simulink model "hw9"  (R2020b)
settings: Solver=ode45  StartTime=0.0  StopTime=15  RelTol=1e-3
undefined symbols (not defined in the file or in its folder): controller, P, trajectory
settings Model: Creator=User  LastModifiedBy=User
settings DataIOCC: SaveFormat=Array  ReturnWorkspaceOutputs=off

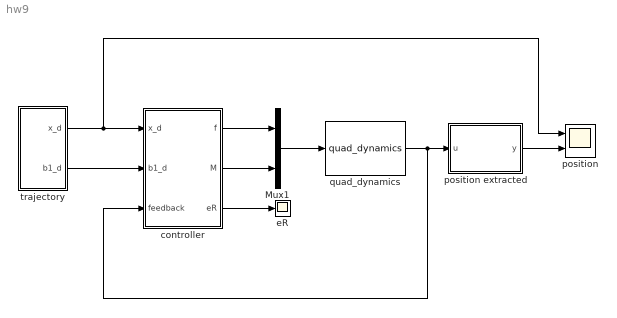
== system hw9 ==
  Mux1 : Mux  Inputs=2
  controller : Subsystem
  eR : Scope
  position : Scope  NumInputPorts=2
  position extracted : MATLAB Function  TreatAsAtomicUnit=on
  quad_dynamics : S-Function  FunctionName=quad_dynamics  Parameters=P  SFunctionDeploymentMode=off  EnableBusSupport=off
  trajectory : Subsystem
  wires:
  Mux1/1 -> quad_dynamics/1
  quad_dynamics/1 -> position extracted/1(u), controller/3(feedback)
  controller/1(f) -> Mux1/1
  controller/2(M) -> Mux1/2
  controller/3(eR) -> eR/1
  trajectory/1(x_d) -> controller/1(x_d), position/1
  trajectory/2(b1_d) -> controller/2(b1_d)
  position extracted/1(y) -> position/2

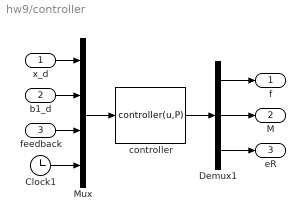
== system hw9/controller ==
  x_d : Inport
  b1_d : Inport  Port=2
  feedback : Inport  Port=3
  Clock1 : Clock
  Demux1 : Demux  Outputs=3
  Mux : Mux
  controller : MATLABFcn  MATLABFcn=controller(u,P)  OutputDimensions=7
  f : Outport  PortDimensions=1
  M : Outport  Port=2  PortDimensions=3
  eR : Outport  Port=3  PortDimensions=3
  wires:
  Demux1/3 -> eR/1
  Clock1/1 -> Mux/4
  b1_d/1 -> Mux/2
  Mux/1 -> controller/1
  controller/1 -> Demux1/1
  x_d/1 -> Mux/1
  Demux1/1 -> f/1
  Demux1/2 -> M/1
  feedback/1 -> Mux/3

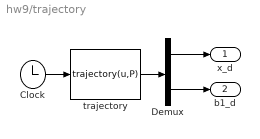
== system hw9/trajectory ==
  Clock : Clock
  Demux : Demux  Outputs=2
  trajectory : MATLABFcn  MATLABFcn=trajectory(u,P)  OutputDimensions=6
  x_d : Outport  PortDimensions=3
  b1_d : Outport  Port=2  PortDimensions=3
  wires:
  trajectory/1 -> Demux/1
  Clock/1 -> trajectory/1
  Demux/1 -> x_d/1
  Demux/2 -> b1_d/1

== matlab function hw9/position extracted ==
  data: u input; y output
function y = fcn(u)

y = u(1:3);
